simulink model "DriveSystemControl"  (R2025b)
settings: Solver=FixedStepAuto  StartTime=0.0  StopTime=Inf  FixedStep=0.001  RelTol=1e-3
PostLoadFcn:
  | if any(exist('dsrtsu_mdlpostloadfcn', 'file') ~= 0), dsrtsu_mdlpostloadfcn('Execute', bdroot); end
InitFcn:
  | , if any(exist('rtifpga_mdlclblib', 'file') ~= 0), rtifpga_mdlclblib('Init', bdroot); end,
  | , if any(exist('dsmpb_private', 'file') ~= 0), dsmpb_private('dsmpb_mdlclblib', 'Init', bdroot); end,
libraries: dsmpblib x2
(part 1 of 11)
PreSaveFcn:
  | , if any(exist('dsmpb_private', 'file') ~= 0), dsmpb_private('dsmpb_mdlclblib', 'PreSave', bdroot); end,
CloseFcn:
  | , if any(exist('dsmpb_private', 'file') ~= 0), dsmpb_private('dsmpb_mdlclblib', 'Close', bdroot); end,
settings Model: DSRTSU_INTERNAL_RTIFPGA=210  DSRTSU_INTERNAL_RTISTBM_VER=23.2  DSMPB_ID_DATA={'1682',struct('BlockId','6bd650a4-7775-4d86-b31a-c7f0cedf2a0a','SignalIds',{{'4d2bf920-403c-42ab-9030-2d9a518b8196','082edb1f-c2f8-4665-87a4-209449b9f104','8d6dcef5-afb5-4d9c-8807-a0699477d6a2','696e1246-c3e5-43ef-a482-7f0d2a84e469','04ea9c71-20d5-491c-a4d1-bb4739dee859','22128026-58a0-4e91-8829-95262852fedc','d869dca5-5dfc-4333-ab53-b3c3e836673b','bfda82c1-d835-4bf2-bc95-aa6ac6e5c40d','fcd5dec7-5735-4e3e-a193-55dd29f5c2ca','a956f46d-fc02-42b2-939f-52e903401f84','ba0c140a-12e2-4a57-8f34-0febb42557d9','6245ff97-b87b-4a0e-8af1-46c4fa2f7fc7','f1293028-aaf4-4ab8-a6f3-082efad6de70','4507e507-dc38-4f83-923d-a5bb48766b92','0dca0241-a3fd-4e55-88f7-513605b5dfba','834a7716-90ef-4018-9252-7e4f04a52069','07042789-bdc2-4e73-a93b-c580a6561b11','74a5c4a2-e22e-4a18-b0cf-773234170c76','a5f8784c-5e53-4949-bb13-5d4dd9b81511','b86019a8-98ec-42d9-9058-f7d65ce9bc5f','188db015-d143-4b34-8c9f-82cb82752dfb','366bfd7b-b2cf-42c2-bb64-21f649b82e17','56ce3dbc-22e3-4204-9c02-f638be6e34b3','c5b56939-1f0a-45a5-9add-669c4c1c62a9','1ad4e223-a404-471e-8730-84e482440c78','9e360379-29d2-4068-a30d-e9271ebfc388','f3f3b8c8-541b-4139-bbd6-2a1bc7723500','32ca3840-ec13-4611-92fa-9ad8c5b7071b','be90de92-4fef-46e1-a0c9-0c40f053aa9c','ba7c0e19-3886-43f1-b27c-69c8bf345196','f9a9b832-0eec-4c32-9774-a7523f529248','e45c8cdb-1cdb-422a-8410-eddd01433567','a79a95c2-bbe1-496d-af6c-65c2c1823672','9c272c79-fd84-4dfb-b005-4b36d7211f30','65dcbbdc-ed0d-47d3-86f1-005a976d3825','8cd805c0-b5b4-4a60-b130-463abf004e7b','a92407c6-04ed-4db1-860b-a24df70c9f97','35edea2a-57c7-420d-aeb3-abf130676984','687fa54f-b94d-448f-a202-370014edac18','b66ac79a-bf51-482c-acbe-a3be231ec044','b493fc17-940e-401a-9995-4d5744c4b1c2','c60e8434-81ec-43b4-bcd5-ce3e34bb3ef5','7ee8398a-2983-4478-ae8d-4ce734bdc1c2','03e69da6-cac7-4a63-87c3-86720c025f4c','48314e02-3fbc-464c-9d90-00d050306e9c','265a4ca5-0bbb-4b38-bb2a-a2c08d6fca1a','83cdc130-4833-4e41-854d-088457fc960a','1416cd66-4df3-4e4c-b187-45789655d8f8','76ad3dbe-0da3-4522-8c5e-5474070f195e','d1ee8ec1-428f-4fb8-83ab-9e5ead026dbd','deea3998-c4d4-4a25-95d6-c2dc6682a3e1','80711744-f146-4f9b-9cd6-5894606187b5','0090809d-e758-4f68-a9f8-fa40a0cf78a6','1ad27d01-33ad-4ad2-8310-e10dd81bfd4f','9ab4187f-c415-4d3b-862e-fd145dc08d78','7ae8cbda-f011-4195-a5ba-479d10d6282b','0d660bf5-2e1c-4ac7-88f9-9e6d591a8ce2','b955299d-9be1-46fa-a0f6-87c26013018a','16df8238-600d-46b5-8355-2ebbc49c0509','0abd2c88-22ad-437b-b7c1-aa302cf4af2e','3837f3e3-7da1-42f6-bed2-e741816623a0','4bcf49d3-b8dd-4420-9e43-0fe41c576929','e41ac73e-d8af-4fcf-96e7-9c28cba251f8','b42dae81-8c8e-4813-bbb5-2f39e8a2b7b0','34b876ad-f245-49b0-b8f8-6ec682069e3e','0c98834c-32a8-41e1-87b3-41f8c1525f50','f30d359b-60ed-4c16-aba3-c6dbef863c96','e9962dc7-0d51-4704-b146-a250d37b715c','f34f35d0-b2c1-4cc5-bb55-4c89c3895b20','3145f379-fcca-4d2e-9002-7bb4c684f0a2','a8df7938-a0d0-4f86-87c4-feca9f5a4372','efaa0a42-a334-4454-a458-d3ac57d5c708','dbdc91b7-596c-417e-aeda-55eb1ac9396d','78b6fff9-505d-4b83-bb79-dadedff90153','7f2d90e7-a6af-4e4b-b796-bf3eabad6eaf','4a0f3a51-4b5d-4063-8cad-a0c21593ff21','e7d20947-3574-4b2a-b795-fb92de4815ed','cdd8f3d4-c4cd-486a-8349-9e1c4ac1a441','555fc523-09f4-4d74-a313-07337e384831','4373e4b1-a00b-4605-aae0-5a5911c23d05','d23501fc-251d-4c29-9393-eaf2c32577b5','aa373a91-4704-4261-9894-f6d5aaf800e2','3c39687b-339c-4d6a-af4c-ad8ecf66fba3','79c9f007-2a19-4611-9c3e-2f6973c0894e','d0c345e3-cd96-4d07-931e-77de4ee97483','49d05b07-b31e-462c-b069-bef8e78563a2','74c9e241-3b39-460a-a122-3519498ceecf','06c0452b-9086-4544-b0ce-aa65222b762b','642581db-1098-4d76-8c8a-ebe9623c49d0','500df3b0-36ad-4b2f-8668-c76bfdb5893f','ff5c5439-2267-4b03-8489-22e5a4527a7a','7f70c939-3038-426d-8a53-a5fc3ecad7a4','f8fd3f50-678d-45a1-90c1-14f8a7ef1f18','f9deea20-af62-4f3c-82be-ea4cdd79cf17','16b84725-3346-447f-9fca-e927ff9b97aa','97121917-7375-4966-a993-77978f9545a8','1ebc6d63-f4c0-4836-b6a8-cf94f8c40ab6','7469b1b6-380b-469a-8ddb-87dc7f11f4f3','fecfe079-c049-493b-8842-df4524f19acf','30157484-4fb3-4404-bc3e-626bd9022609','90c29c88-b6bb-4df2-ae3d-dab8302c7e72','891d6475-5f7e-40a7-80d0-0faf1364944e','ce6e7f2b-cb3e-424a-8b0f-3ef4d0f778c2','80a6d053-d3c4-458c-bdb4-e8d2f1d58b6f','f5d19550-38c6-4cdf-9d3f-c7ff2c4edf42','8679dab3-89b2-4b8c-972e-adb9b0956be1','6d1a9255-21ca-4408-acd5-50988fe8969c','51dc251d-1242-4cb7-b761-fee981f77b9c','62132aa5-934d-47a4-aef4-8ce71be6cb39','54be5f98-a02d-4a55-91b7-e0eb3db5b29d','42ef34f8-decd-4543-af15-90924bc8905d','c9efaf1f-4082-4ddc-8e56-c65a017542cc','48f0e1b9-c04a-4854-91c0-35f6c82faf8a','1f3eded7-d459-4795-8dad-7f0dd28c087c','8099e6fc-762a-4979-bd34-a91a25cd7676','3527f9bc-ed9d-4dd1-84d3-55a707f8be99','1bcf277f-c8d2-40a1-8315-1aa473223f2e','fa6c0776-aac4-48f3-9396-764daca02d47','8387cd85-a5c1-4904-876d-f704e78f2c62','387533fb-e797-4ede-99ca-d4db8180f387','1c4c3dd9-5635-471c-935b-5eec6f46986b','e459a777-4251-4b7d-893b-90ad6317f334','17defb02-61c3-4cac-8487-2282098c4bad','962847d2-edea-4051-af97-97b08626d83a','42a313ce-3314-452b-ad2f-f3a113c22cb3','75d3fcec-c027-4b3d-bb70-d22582f25c13','fd2a2273-8951-47ed-835b-df74cc3ba1c6','bddf05ea-74a8-4d40-87a5-fa5bd6bdf322','2fed9884-dfc8-4a84-ae8f-f244653a61d3','9c3f887d-4bcb-4f6c-8796-249e51e8bb68','959b4826-76d3-4fc3-a833-b714fc953f9d','e7570022-f6c4-4e8b-a861-bb6066ff821c','b83962a3-0493-45cc-9bff-babc028f8765','1c359195-adf3-4f7a-973a-0a2c48996ddd','b2deb9fa-fd3d-4fdf-ad07-8606d6acaf75','88712765-a778-4989-9373-32db34a7e96d','3e70b9cd-2371-4f82-b9f6-12ee1415d8b9','7d58b90d-1048-43eb-af67-3288cd86feb8','01444fd3-9787-4cba-b0a2-4888be12992c','9db5b754-e9ba-4b7f-8ca9-81a8af447387','bb3c8869-bfbf-4ea7-bad8-83df8fbc8f98','5ed3fec2-9b08-4d98-a442-0ce35e27cc88','f0712c27-75e9-4f86-b8a8-ba457760ea16','5358583b-35c4-47cb-89a8-767083e8d807','023bdaf1-a030-43b0-9700-cb477693c83b','8dd5c8ed-0ddc-4ed2-bc0d-28f253869c67','9c9da58c-c166-4097-b5fa-7ea9d6f6695e','dfb39263-9b69-4474-b81a-c4d30d70140e','ccc703b7-f3e5-4cb4-b5b1-83ba1caa6f6a','52fe69e6-650a-4d77-a362-9076dc4ac840','565d162d-d064-4790-89b4-314f96e2621f','0ccdfb67-d94d-4e1e-b614-260b93448974','f50cce07-cf3e-4a8b-9eeb-7142a34334e0','11b69825-057c-43f4-9a52-cb286eff8a67','d1d74e82-881a-4d6a-99e4-eba536a09dfb','2e87cb75-a918-43cf-9a95-f0e5eace9422','1fdda0ec-b29c-4da8-a1ff-2f579d2fb1fd','4e5165ab-f934-4af7-aaca-f8701864098d','3f448d55-1dba-4c7a-9308-f0598cb6fa01','afead3bb-0504-4425-9c8e-ad2a378fa778','2fc7a59c-fc8f-4fcc-b5d5-65e69e44638e','435b3590-798d-4988-8dc0-ae2dfe9fa36c','4ca3d702-9700-4467-8bc0-5ddda41c78d0','744d85cd-5be3-4dea-a3a6-0064f59251b8','d914b334-6d5d-479c-97bf-c042d637b381','c67e1c2a-0e05-4b9b-9862-c5b24a3e52b1','a8bbb01d-de2b-48ab-82c1-4010a7c7741a','69f9f471-42d7-4015-b2e7-5a903b3d223c','6865599d-3bab-436e-b378-8a6065ccd8af','228dfb07-2cdc-48a2-beda-1fa90fce3f7b','a8fc89ea-6636-4534-9ba5-5ff0ee9f268a','f6fda9d6-d985-4630-b1e0-efbab3a7f748','0aa2a0fb-9f0d-4277-83e4-df9dffda4f6b','045875c7-e102-4128-bbe5-63fa3b05832c','cb5cb840-8ae6-4f96-ada0-a55d4e4d95ce','9c81d51c-ab73-4745-9266-3acf8ac06247','e4bfa2cb-97c3-4fbb-8dd7-6355edc7a0f8','713cd20a-a3f2-4ba6-88e8-80a6ce871d68','66ee43ba-5bdc-41d6-857a-0f6935ab8e39','13292625-30bc-4997-9e6b-497de6cb1190','acd60d88-547f-4390-beef-35e3f10afbf2','06cf514c-8df1-40fb-a85f-61544231c781','3335d807-6857-4b5d-8713-cbb5aeb56245','8263c7fb-fc40-4678-904b-dfada2e27b25','b93b61c6-d2bf-43d9-8ed3-0ecb89309517','ea82cabc-8a5a-46b8-bb1c-22b49babb383','5fa73027-c1dd-4fb2-892f-8bca7fb9b94a','82f31a19-c2c5-4607-989f-7586beda9dad','d76ef0e8-d179-47a1-8ca8-dbdf90b2a140','d501bdd8-1a03-4416-88e3-6351e0c46002','993ca02b-e763-4089-9f78-884932ce66de','b96a593d-cca9-438f-bdb3-641fabf17218','7558054b-8ba6-4fa7-8754-04b15e84ee6a','d7bd8e5d-2ff7-4dd2-bebf-c2bdb021b32a','94aa826e-0097-41c9-a4e0-cc5dd6c74607','c03f5656-a05e-4c14-bdf0-c421ae208cbf','49f7be12-6ad8-46f0-8a68-95fadeb165e7','2ae149b9-9578-4644-b4ce-ddf2e155d9f1','d6938736-adca-47f8-89a4-0915447342c1','cbd99736-1323-4b52-9170-d05d706ca95d','917397c2-3823-4180-b1c4-179169db1045','bbd7391c-67cd-411e-b5f9-3ac9dbfdb24c','7dfd2c75-dced-4705-a5e9-2a2a2d4c1ed2','85c981e9-72f2-44e5-8699-e41a8b3df25c','dd72fa7b-e733-4fbc-af40-78ba69e4bb53','bc0cf145-a984-4d25-894e-5a8c07d2e8b6','8918bd77-24ca-406d-81b0-9f0f71eaa5b3','aaf49a73-eadb-4988-9e1c-1f4687a0c5a7','88db5271-3e64-488e-8998-db478282d9d1','5d6ab81c-a00a-4771-beea-f142fc88acd1','46b0c3f9-c34c-4232-a295-52e3606efea1','e47f8773-eb71-4d5b-973a-54a731f551ff','085e50a1-1138-45fc-a57d-5399a02ce4d5','a344b347-226e-45f1-b0bf-9cc140041033','90f24455-1319-42d1-b784-e412caf3a4ac','e2e9fe19-b98b-4af6-85dd-ec4afb81798f','2eaa310f-fafb-4421-953b-c578c89e6b62','893ed9ba-a67f-4d2d-8513-ab44da56141a','7611d5a1-03f3-4973-90a7-64cf3237b486','3ae57e55-9b3d-409b-a7f6-de24e0e54807','c32b3135-c5b2-4e6d-a033-f1d56d13b3aa','0df06ca8-5346-484a-a408-79d691d949a7','5c9a9b92-4eb5-40d4-bb24-32f8ca60fbf2','ba01591a-99ca-4f3a-a480-0b29c9493ed5','2be9e2fb-4140-4463-b738-10266a35bf3a','615d2e04-5e5c-4153-a094-c8ec447c30d3','55a69a7e-6023-43c3-b133-bb865a033567','f9bc7cf0-32cf-437f-b915-b91298c7960c','43dc8092-f3fe-4614-a6e8-4088139e8bd1','b235cb9b-c3a2-41a2-85b6-9bddb082eec2','a64dedfb-6ee9-4a4f-ace2-09eb0ee433c8','f640fa21-cb84-4772-a512-7da12fd1a438','40fb2d7b-d7ac-40c8-98c5-b3c8732c033c','687755fa-7e4b-4908-a181-5af136a86154','4529d789-9ef9-4983-8bf6-7cf797bb40d9','dc2e8884-fa4b-4ff6-8f58-4e5e018f2bfb','3f263054-263a-4fa0-8fd9-a8cfe8c07787','0cbdf9b6-3173-46d3-aa7f-08b1c97744df','62cce852-fba3-40b3-93d8-491895877bec','cb4b3a9d-4f04-46df-b3d8-4697ff999350','ce6668e8-c0e7-495f-b37a-2f268e9d531d','85245983-2e26-48c5-a724-bde71d713a38','4df0109a-d5c5-43cb-8227-843af0b156a3','7ebc83d5-ad1c-48ce-a6e1-c6b0ab638476','5f64f960-7181-4cb4-9b5e-fc8b5295f45d','41fd1b04-a66a-4364-b9db-6aa7bfff160b','ea3e3dd4-c3d1-458d-adee-604f83a1ee04','af992076-6822-4ada-80e3-ab6dbc5d9d4a','c98eccdb-4c6c-4db6-acb3-c038b733bfac','ffdc664f-aa83-4dff-8e24-22198390c623','8887eef6-f5be-493f-8399-9f81aef6b3fe','a3528d63-51b7-4ac5-9b90-dce70b5af3b6','ad3f5d80-5856-4ce3-b36d-eed9eaa3efea','00c26369-2aa0-4cad-a24a-1697bf176f97','31b89546-fd4c-44d9-b714-de647cfcd9b3','7c80e928-01e1-49a5-96ea-91f6f9f61a2b','ccdaa406-b4d2-4ff3-a2f5-cf4e1644c887','2ae4ebd2-73d2-454a-a6ee-b929d7cd9a6f','4c7480a6-67ab-4b7d-b1cb-8e892c1369c4','b0d7b28d-4bed-415f-aa8b-6ae9d75690f6','e8908c6c-abca-4b58-a419-5e9c3e02e2e4','add271c7-7c49-4768-ba7f-7043464bb221','2470019e-d8f7-421d-8a57-7a385a3d6780','6f5bb2a7-60f4-42ab-9dd5-034207f55142','f911aee7-c5e8-4e2c-83c8-defc6b1f5653','38f16109-5af3-484d-a1aa-bbf2744b3099','c49c3c33-831b-40e5-8613-00f9b6836ba5','9f2e7427-64dd-478e-907e-1bb111fb7334','7eb8d7bd-f8e4-4dcb-b36f-c37d8c5e15d7','1b3ca147-0424-4ed3-ac05-fd4715a7f247','3b9bf52a-173b-484d-896b-4eecbff99b70','5f5a62bf-9d15-40da-812a-293289ce1b56','6d87a8f2-96ff-4bc1-bb1a-706893b7af83','eb9f571a-4bfc-45bc-aafa-e339e141cb62','b024688b-8b72-4461-b70a-62d23389103e','d6ced81e-c41f-47a0-9c81-f2b18ea1e2b6','7563f16e-4634-4ab8-aeba-4bc6beebcdfe','4ab347d0-3229-43f8-95c0-de0104dcaba7','2f90c9b2-549f-4e38-b380-4a5c8bc2e0b6','504b50c9-25bd-4815-ab13-0da8bdb25c30','3c742c5c-b08c-417d-8795-0984c0333b9b','b5e99845-aa43-4fde-a8a3-234b17d30c19','59c0f048-8280-4d2b-bf7b-44fdeb4866d2','824bc859-b681-41fc-81b4-03ccbbbc3a8a','77731384-ba52-458b-8862-31b6aa2e9195','38fee5a6-2ec2-4c23-9671-ad9db19ef98c','81f68cdd-f880-4766-9962-450b510dca2c','e36217fa-72f4-424f-a1ba-26c56e3b9a0d','f68425fd-7a5e-4827-9af1-d350a4f38e36','6ea8ee41-3bc0-4644-ac9b-1f597c99a9c7','ab82a394-39ff-41de-a9f7-cb5ef0534498','4f10cdaa-3e15-43d3-8f79-6b8dbc1a7a38','522704e6-d62e-42bf-ba3e-a117b8a59b5b','e0a877d8-8871-462e-8559-bba47ce65c7a','1046ff0a-d910-4642-a4a6-c04fe5f52276','6aa983d4-51f3-487a-ab56-90ed78ca5151','24efa16d-19e5-44da-88be-4fe7ecef26c0','81f68b0c-bdf1-4e45-bfd7-e55567c3dc04','4116bf02-b21b-4eb1-adf6-3e3c0dd2eaf9','6066ab77-e5c9-4ec5-b285-858f37379a7b'}}),'2',struct('BlockId','fdeae165-f251-4e82-b59a-3c43838b8ed1','SignalIds',{{'de8b44b4-5422-44ef-8723-6bdca849999c','7b06e3d2-1eb0-49de-940b-866532a21950','74468e4d-ce7b-4114-abcc-ff4ed516802e','09b3dc75-925f-4156-8fba-f27b88531e74','0d939a05-4c0b-4c2f-ac9f-c224cb75ad55','61fa365a-d2fa-494d-9414-3405a4ce6d0a','ce00d0ab-86c1-45f0-9867-9a3821da710b','f31fc571-c561-49d2-9f91-922cc8d9329e','0a751642-ad47-47ce-8c4c-87b9c8bace46','b29db070-bfb7-44ce-bbb4-dac7cc04df61','a0b6132c-c02b-4ec6-93db-95c6745521da','d513a490-61fc-40bb-9b15-a9912397190f','5d11f126-fe30-4254-9ca3-30fe71e76f3c','48fd1300-cd08-4009-87f3-302b4ebf7052','66062813-008c-473c-8e52-deb424770f9c','e0ce1efa-3209-46ec-8e83-f1336c285641','2f9e3794-b3da-4bfa-984d-30fae498b990','83f662e2-91a8-4716-96cc-1d31ae3903e5','ed013d79-9480-43d1-adbb-ef641568d862','245c77d0-9eeb-4469-8ad7-ddd6cca0bdc7','109a2097-3c50-43cf-b22c-e32e4f0d4b16','5c8654f8-c4bf-4464-ac59-550e46dfbe36','053ac246-b2f3-4500-b8dd-d680c86b03fd','7a8feb55-fc6b-4238-91ea-6e4b4e7558e7','d016b082-1aa2-4773-a812-75518ae20876','8789bb0c-d99b-4489-8c7e-d41abab79294','1b300131-2ece-46a4-ae79-1cd046174832','27185aed-9b16-464a-8e1f-1ad039b150d2','dc5d8b8b-96a3-416c-8c53-f6439024a3f2','53d4b546-2e80-41d7-99aa-9cd9e4df08a4','9d062d5d-415c-4501-a210-a13c9dc09661','f2802ce9-2474-405f-b2fa-9033a0c19371','c35b0d99-e3ee-4fe3-adc4-cd41e3c76d9c','2cf185fc-7a78-491b-bce7-d7593e39c21d','9f8b6ee8-2ea5-4f6f-8f38-bdc62e5a5876','a5d2abe3-156f-45fc-8d82-5f1c828eee06','60f59446-fa5c-4a1a-9f1b-2da327279d46','8f11fc00-2091-4a34-8c6b-ba6a227f3728','b48f3cb0-dfeb-42bf-83a7-6d2e2c9f28cd','df21d149-9261-4d80-ab0f-bced706a3188','b57734b1-8e0a-44d2-9318-0d83da79d543','6faafaed-af4e-43d7-9806-29c97c255c6c','233beed0-43f0-452c-aa34-82cfbd4d48ac','465d0d2b-5ee6-4937-9a44-db7d6bb66479','bc7ff652-41f2-4daf-879a-5b2921b89016','7c3d8010-5c5c-40e3-b1ae-5692f53c86e8','9666030d-3a17-4d78-a81f-8b72e34b0b66','0c513926-8004-44fa-98f3-f956c2aab0fa','9166d83e-c4c2-48fd-b219-1b7c9d6557b4','cc755fdb-0eae-43d7-8eb6-4ca175b2ce2f','bc3a07b2-a619-4c81-b3f8-feb17cfbcce2','4e564945-a3a3-43c1-841e-93b5d941de79','09af9a1a-9f3a-490d-a22b-1e244a520192','0fee6cdc-ddd9-4de0-9902-dc7f9d2495d1','cba0aac5-3610-40ba-95e7-3214ee2eb255','d957393b-e4d4-466c-8db6-61d28ec803fb','d8a45f3c-0399-4f7b-965f-ebd23a625cc9','74696636-2799-47bd-b6c3-7bbc02a97467','32df2c93-5398-4279-82d2-8ad464d076a6','45e3dc24-a076-40c8-938b-1c108a74d5d1','735a660d-7436-48bb-be5b-89cc0edc3658','10980fb2-941a-41b9-8141-8bdc6fe828f5','4d8ae5ff-336c-4f2e-bd45-d0e31a4eaae7','955c6127-9ce1-461a-b6d7-5551c6febfc7','522dff20-4a47-4e98-8115-6a9305e6acfc','c2400870-07cd-4018-a99e-23e7da5108e1','75701347-3308-45ba-bfb0-7d593a167a16','5b1f0e37-5598-4687-9cc3-c7f1d3495d80','b355af3f-48f3-42fd-9da3-9c53df86dd66','84090b07-4cf6-4aa5-a80d-19288670be82','2e4363a3-2349-4f09-84e5-00ca8294403d','468f28a3-7f8d-4e9a-98ba-22c9251e9022','b9fa48eb-8926-4a45-9a4c-2df5a61da293','2e70f4ff-309e-40ea-bc25-5b9c3b09de05','19980cf7-9fa9-4830-9d3b-932aceb94898','7a57d7ac-979c-41f6-a94b-75fe1c9dc488','4817d061-27af-40f7-bb85-993186cfface','7bff44ec-3940-4df6-906b-5ebb1cd609eb','4da95aff-fd17-4a13-ad0f-df6500b75cb9','67be5fde-06d3-4a91-b8a8-8f5a874bffb8','aed8f512-8d75-49d8-97ba-7cdcaa4ec92b','2081fd6c-66db-4b19-9031-a92910431a1b','9b269a33-7c5f-4e87-8838-4dbd5e03684f','ead4c6b7-092f-4771-98e3-f228bc0df61e','09d15870-e3f7-4818-9260-8cbd79fc4934','e1c4632d-8d1d-435e-9cc2-1a1d7cee0134','be392e74-2c9a-4303-8deb-b6ebecb41bb2','3d160701-0a0b-4a9e-911d-7e5f1dca8da1','a10638db-8be5-418f-90c3-8a20284ef010','46845510-bea5-47b6-a852-33e47d9a4bbb','1096f6c8-0051-4daa-93bd-08ee419c3d60','e40a998f-3667-404e-a490-3cb0f0305e64','de91afbc-364c-4d90-8544-7e581d5e6036','977c9308-4cf7-4ef9-9655-eecccd4e37ea','8135e324-4d45-41aa-9edd-83d48a353d7e','cff61663-a888-46ad-8242-c681d34892b0','c59df38c-1b9a-420d-b5b6-7b02e9f30d14','8c3f161a-015a-4ad0-b6cb-70b756673a80','ddea31d3-517e-4adf-adc9-8410399cc30c','2ac0e3f2-35de-45a3-97da-d45fd9866c6a','5cf57e47-2f74-4e53-be91-f6f7c6319c02','e6ebc12b-6c7e-4c2d-89bd-1e13fbfe96c1','bc7606f6-bdc9-4d7a-a134-d3cf085f353e','652e12db-6510-47c5-9cee-3289bf08fb81','32dcee06-8d73-4567-a14e-b4948d0c7c57','be60a994-383f-43e0-a6a8-e25bbfdd91de','990e0621-b375-4e80-9796-4e4ace91b209','bdd403ee-ec2d-44e3-afc1-6fe71c0e26eb','81afed3e-a265-49a6-b3ad-6cabe8f91ecb','0a983437-82e0-4732-bd97-f41efdc05314','5e76d710-901b-476f-954c-5430facedaca','3be0e1ca-d6bc-4bd5-b8d4-50e1289b089b','c504ba16-f24b-4614-ae03-4e76a49f7adf','932897a8-81cb-498b-bb33-ea7d7b0238c4','f2665638-91ea-466d-97d5-d52c7b16d6d5','043e2de2-04fe-4e3b-b0c6-5ddfa18c1d18','8f3c1a59-5ef2-4f4c-9629-a0484fad656d','2f116884-4cba-439c-85c4-3547126edc4f','dd612bf9-7c57-4164-a759-b3de7707c278','4b187830-e30c-4f4a-aa7e-32f00e661252','fbf0f747-84c1-435a-8184-a67b43aa0379','b3a9ccbd-8fd1-4c1d-8fd1-4362dcc93e97','f6f40c37-99f4-46df-b3d0-72f5d2793989','1ab4b575-6948-4afe-9774-20425c1a8951','07728060-6cc8-4bf9-8b9b-5f5596c45ab9','ac6d2f26-54c5-4a67-bbc5-680bf04eb5d8','57e3ba4b-9507-4f5e-8ed9-618e71123933','de0c428b-5ba9-4ad2-8078-206528c55396','afa35936-e8ea-4a9c-a9cd-c56e07d7689f','0bb38e01-f1da-40c0-a9e9-6de8e14cc2c0','47a2144d-6aeb-4d86-bd89-49b5844ec041','65b96597-0582-4f2a-86b1-26455202c868','ff25c3aa-f958-42b6-9e59-f5a026dff9f4','2905a61d-4f68-4d1f-978a-afc6c65f5737','3a41da83-63a1-46f9-a952-8b9af7794f2c','d5d01b3c-f436-4b5b-82c1-142de6ff27ad','447ff66a-31ed-4fbf-aa67-6305ea65f05d','278a5484-cd16-47b1-b117-efe68225702b','5c3ba11a-3515-4c0e-868c-f2cc44378a3c','b8a1b769-223e-491b-a256-ec5a6f28fef2','a1d96fe5-c3ba-4a23-901f-02173da89a20','4b9770e1-7a75-45a9-8578-d72916c107a1','c27f1bab-f8f0-4a84-a154-2f177810a256','476fd6db-b212-4592-9a4a-c22e7d6b84eb','2e4e1afb-2734-4baf-97ad-0100df7323f2','0210cdd7-b46c-4281-9a52-c0544873f54b','56144df2-637e-456a-ab58-3430fca16b2a','dbfd772d-d01c-48e7-aa6b-9e74b92c9a19','61bfcd02-3e15-4f08-9ad6-0a80ec366a4a','d76c8ffb-b399-43d4-bd45-30aa88148c11','3e57bbde-eeef-433a-9c1b-4ff6b243bcb8','ecfc6bcf-12a2-45ec-9ee5-91807b0ae174','32c4bb39-d309-4ad3-8e1d-d33ca5046e76','7846b9f8-0593-4e8e-8339-59be79bb9e44','8c280d6c-ccc3-41c2-aefc-75b0b983aba1','b8245033-a011-4e70-b677-32c48ba319bf','1806b3b9-7fa6-4329-aad0-38a4cc9c3a0d','3cc78dfb-37ad-432b-afb6-10d890ce3613','a580af44-a49f-48a6-a1e2-bc7cd1a7761f','7eed13f3-b9fe-4789-a07b-330ca8d35faa','93f81d31-f14f-4bc3-a614-8c0b4085b5d9','73f1cef2-8057-48cc-aa1d-ac1323c43fb1','5db861ba-aaf6-4c67-b7b9-bb818399091e','e7ee0ff6-14e9-40c0-8ac9-4df9f11a6683','bb839128-0c40-46e1-9127-4d997c649eba','f5e2cee2-6f4a-4069-8698-01e792f15bf5','040c843c-0881-46b9-8ccd-7fa67e5a8526','a96a21de-c0f1-480e-abf4-c62a0a739262','0b64d65c-92c7-41a8-8fc9-f7ccb397cb14','9f05ec84-b3f2-483d-a38f-5b354dd2cf57','480e317a-2597-44d3-8213-8e3d613866f8','24b4c2cd-7e82-4de1-a48b-a7c044870a20','81966acd-aa96-48c8-8018-a9545624582b','2c2af29c-d3e1-41db-ba0a-1f865aefb512','7c0b55f8-ea91-4077-bd8c-cc6bfb22dedb','85588d04-f050-4133-a21f-7692b804045d','107279e5-4394-4265-ab5c-29a6df39d858','10acbf4c-799c-4e13-a154-848ef2cf3d06','10dad0d3-d666-4179-8b68-aef958647a07','5b8c799a-4e30-49c4-8ab6-ecbb26938cc1','fbca3a12-5897-4410-bccd-82575ad7b2ff','529fcb8f-b307-4514-9620-e1b2c833d4e3','067906f9-22eb-46e7-b210-dcfd1b0b7eca','1d8d3c3c-58bf-4331-b897-e4eafaa5b8dc','03c82172-e26e-4cf4-90d5-2195b8000227','655349db-53c1-47fe-9446-0ee68c443f65','2e018f93-4293-4832-b3cc-e4db5589e226','147eea70-4f58-44d2-a21e-44109cd1bcb5','66945845-1ce9-496f-9a4f-ffe4e51837b5','499c724f-c37f-48ba-a1f4-28ac52df7ea5','b6794d06-edc0-4606-a429-57aabafc5ce1','cbc1cb93-8de4-4a68-81da-eeb179512be7','63184478-25f8-4e5c-96ab-f649643fc6dc','1d4d4c13-8d7a-43a7-82fa-8823d056fb47','a7010fba-113f-4abb-934f-a1d598db6650','d60151f6-e2bb-44d0-97f5-b9a6b446749d','c6e18689-1cfb-4099-8655-dbeea30a1865','bedecf49-055c-4280-a56f-d9cae2990382','4f1ce29b-2afe-4ca7-9a57-22a60e90ba30','94c28d1c-303a-4304-ac13-44f231e8e68d','59ce40cd-53ee-4803-9e0d-e5ea17f4cff9','9a5167ea-a9ce-4bae-83fb-71637c8cd1ab','7e45628f-bf64-4921-a76f-4f974fb9fe40','9b3f5dfe-9eb7-4a31-abd0-56a510178dc1','75cf1272-a273-4083-a26d-3fea507291ff','0fc378fb-3d88-4771-a129-17a736f54c2c','b241270b-68f3-40d1-9491-2ee7e36148c0','a769bb7d-1d78-4ec8-a3f6-bd492bf63750','576bc8fc-bebc-439e-b4c8-3086d4f4d778','e0b9c0e4-0e15-41c4-a55a-5c8af835c3a8','7ce844ea-f31e-426c-bdfc-26589907def4','a94b0dab-8855-4ff6-98fa-d5b0fa5f7cbf','5e2634c0-e882-44cb-af7e-da85caa29e0c','2f4703e9-16b6-412e-ae5a-daa5147d0e99','9df47e29-c871-435f-b6d7-9bc6a45234c3','0b7e4c49-dfb8-4e4c-be51-2aa0924f5d0e','30848cd8-b7c2-40bb-88e6-af4923ef4463','803dbca7-d9d6-46f5-9b8a-1f5dcadc40ab','8276e255-0345-4bba-984f-28286ab88662','2e1dc2d9-db99-4c3c-94a2-1d1accf58fd4','bfbfcfe5-c032-4f33-98b9-f08a142d4b3d','2c76a0a7-75da-418b-92b2-b4abbe9d7631','3ee28d08-8b83-4b2f-add7-3a450c57c357','edc7a7e5-1201-4829-a751-479dd5624d67','22440fc5-d4b1-4a38-af36-e4aebaff63cd','4e8cf599-944e-4d81-a460-d342d6d656bb','67187d27-f8ae-4e07-bd5c-8f8e68ce107f','31813405-b512-43d5-a107-22f42c7efcdf','12a3c7b2-0ef8-42ea-b257-433533060951','94d7e6c9-1a49-4644-9642-7d23adffa9a5','41af8ef3-86e3-4f2a-8ccd-b49473830aff','291e49a3-cb15-4225-bd5f-cf812338c3a6','6ef9c6c9-46a8-48d5-8bb0-804c08aa3838','f53d4411-762d-4469-9b83-26ad48e1d186','2c14f202-fa96-49c7-af6e-229620f8a5f6','e161c16d-c154-41bc-8151-bcd304adeae2','e491f51a-aabc-4e34-b99f-32892cce09eb','6f3ced98-1f32-4227-af27-721b08ccae0d','ab338563-17fe-423e-8c7f-6671bd4ae339','876cb448-710e-44b3-9042-04655f65fd81','cb280c1a-7567-4d63-bd86-5fd0ef4de71a','63911ff8-0890-4322-b749-398c434f08e7','14f15975-9622-4b8b-aecc-e014706ce072','cd17c7e4-da5e-4b1c-a54e-d5ac94ae44a0','ef0a9bb9-bb14-42f0-b05f-1781a6e36247','3c31f4d8-11fa-4b27-8a14-0f9f31a0fa3f','e3c1f15c-637d-4a17-87d7-3c6a9b240052','5c6aaa89-13e1-478b-97af-dfaf5001a808','6fdc1402-2e8d-4478-8717-65c6f9116fd5','780aac3f-8a49-4430-8e9e-9e74d81ed1b2','fc85fb86-64ec-459d-b0cf-9cd95bcb9d60','6db658d6-cb72-47b6-aebc-ea68633b9036','b95c7cc0-dbcd-4537-ba1b-7781767d1e14','237d60a0-3e9b-4996-8830-289ba11d6b9b','455bc271-368f-450c-a7f1-f31883bec460','47cbee84-623f-4332-834c-fd99b86fb540','79fb1432-8cf2-4971-985d-57ef54e4908c','c2795267-1999-41fd-9b63-66902f5c0d82','5f34848a-10a8-4ce4-acd7-952ff817484b','e0ae91eb-2846-4fb5-9dbd-2d8856d56dfe','fdf3638c-77a6-4082-a4be-ef4b62e07f08','7c29b997-b3b3-443f-8fae-3f9f9e1753ee','7d413e90-90be-471e-af49-f54a2a95f939','8e236231-9214-48f9-a541-987c1d5b7579','bab97780-9874-4de6-8d70-c4bd6bd05cf0','9d793aea-5988-47de-890a-db90f1c3707c','9c125b00-d52e-4fa6-8ccc-1e4806ac683f','81e509fa-0d6f-448b-8368-fb1571c0bb70','80910651-8b2b-4abc-b522-3774286ff664','17d82bd2-7fa6-49ae-acdd-a3900593374c','875b3e42-7eb5-4f2e-9c6e-b67881d72b2b','5430afc4-d9b2-472a-b6a6-0ca88bce53ff','b71a725d-0a81-4362-8dbc-22226aae632c','ce907282-1c16-482b-80bf-a6d1fed3b919','f8b9c411-1d29-4f10-a55d-9850703d42f6','15382d29-5d33-4cdb-bb58-eba90d4ab5fc','87566085-81c6-4f92-9d59-7bc4afcdb0fe','a1b5ca3d-8df0-4d46-8c07-4d1ae1986830','a4000a69-fb31-4fc4-ac92-d20106dfcf1e','bc9a8452-3b12-43e7-b29e-2048af94c161','b64bf5c9-86bc-4428-881d-5e6eb60cd202','c6ff0695-a359-4ced-9d27-40b774cacb7e','ed431a80-fd0c-404c-9126-2b84d01145b2','86d73309-2c10-4464-a04e-4b7ff154f585','923864f6-60cd-409d-96e8-3cd88239526f','394a4075-5ab2-4698-93a8-830edee76a4d'}})}  Creator=MURTI
settings OptimizationCC: BlockReduction=off  ConditionallyExecuteInputs=off  OptimizeBlockIOStorage=off  BufferReuse=off
settings DebuggingCC: TasksWithSamePriorityMsg=none
settings HardwareCC: ProdBitPerLong=64.0  ProdLargestAtomicInteger=Integer  ProdWordSize=32.0  ProdLongLongMode=on  ProdHWDeviceType=Custom Processor->Custom
settings ModelReferenceCC: EnableParallelModelReferenceBuilds=on
settings RTWCC: SystemTargetFile=dsrt.tlc  GenCodeOnly=on  MakeCommand=make_dsrt  TemplateMakefile=dsrt_default_tmf  RTWVerbose=off  GPUComputeCapability=3.5  Description=dSPACE Target DSRT - Generates SIC files for import by ConfigurationDesk and VEOS. Provides code generation for Simulink models imported in ConfigurationDesk.
settings STFCustomTargetCC: SystemTargetFile=dsrt.tlc  TargetLangStandard=C99 (ISO)  ParMdlRefBuildCompliant=on  ConcurrentExecutionCompliant=off  GRTInterface=off  DSTargetArchitecture=Default  VDFType=TRC  TRCOnlyGlobals=off  TRCGenerateLabels=off  TRCGenerateVirtualBlocks=off  TRCGenerateStates=off  TRCGenerateDerivatives=off  TRCGenerateParamValues=off  TRCIsOmitVdOn=on
settings GRTTargetCC: CompOptLevelCompliant=off  ConcurrentExecutionCompliant=off  CombineOutputUpdateFcns=off  MatFileLogging=off  CPPClassGenCompliant=off  UseToolchainInfoCompliant=off

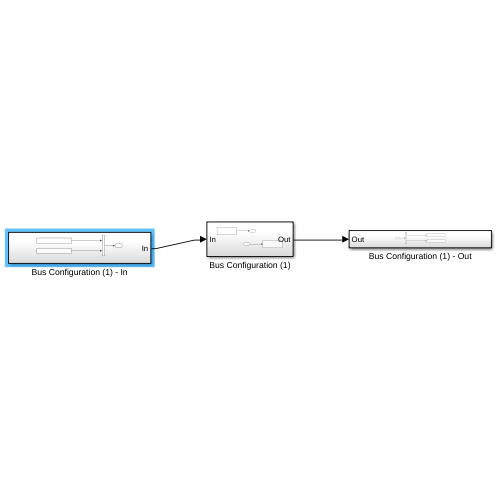
[thumbnail: Simulink's stored preview of the top-level diagram]
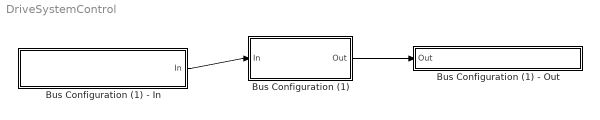
== system DriveSystemControl ==
  Bus Configuration (1) : Subsystem
  Bus Configuration (1) - In : Subsystem
  Bus Configuration (1) - Out : Subsystem
  wires:
  Bus Configuration (1)/1(Out) -> Bus Configuration (1) - Out/1(Out)
  Bus Configuration (1) - In/1(In) -> Bus Configuration (1)/1(In)

== system DriveSystemControl/Bus Configuration (1) ==
  In : Inport
  Bus Configuration (1)_In : dsmpblib/Data Inport  Priority=10000
      settings: SourceProductName=dSPACE Model Interface Package for Simulink (MIPS)
  Bus Configuration (1)_Out : dsmpblib/Data Outport  Priority=-10000
      settings: SourceProductName=dSPACE Model Interface Package for Simulink (MIPS)
  Out : Outport
  wires:
  Bus Configuration (1)_In/1 -> Out/1
  In/1 -> Bus Configuration (1)_Out/1

== system DriveSystemControl/Bus Configuration (1) - In ==
  Manipulation : Subsystem
  Simulated ECUs : Subsystem
  _In_ : BusCreator  Inputs=2
  In : Outport
  wires:
  _In_/1 -> In/1  "In"
  Simulated ECUs/1(Simulated ECUs) -> _In_/1  "Simulated ECUs"
  Manipulation/1(Manipulation) -> _In_/2  "Manipulation"

== system DriveSystemControl/Bus Configuration (1) - Out ==
  Out : Inport
  Manipulation : Subsystem
  Simulated ECUs : Subsystem
  _Out_ : BusSelector  OutputSignals=Simulated ECUs,Manipulation
  wires:
  Out/1 -> _Out_/1  "Out"
  _Out_/1 -> Simulated ECUs/1(Simulated ECUs)  "<Simulated ECUs>"
  _Out_/2 -> Manipulation/1(Manipulation)  "<Manipulation>"

== system DriveSystemControl/Bus Configuration (1) - In/Manipulation ==
  _Manipulation_ : BusCreator  Inputs=1
  gitam Controller CAN File 08082024 : Subsystem
  Manipulation : Outport
  wires:
  _Manipulation_/1 -> Manipulation/1  "Manipulation"
  gitam Controller CAN File 08082024/1(gitam Controller CAN File 08082024) -> _Manipulation_/1  "gitam Controller CAN File 08082024"

== system DriveSystemControl/Bus Configuration (1) - In/Simulated ECUs ==
  _Simulated ECUs_ : BusCreator  Inputs=1
  gitam Controller CAN File 08082024 : Subsystem
  Simulated ECUs : Outport
  wires:
  _Simulated ECUs_/1 -> Simulated ECUs/1  "Simulated ECUs"
  gitam Controller CAN File 08082024/1(gitam Controller CAN File 08082024) -> _Simulated ECUs_/1  "gitam Controller CAN File 08082024"

== system DriveSystemControl/Bus Configuration (1) - Out/Manipulation ==
  Manipulation : Inport
  _Manipulation_ : BusSelector  OutputSignals=Virya Controller CAN File 08082024
  gitam Controller CAN File 08082024 : Subsystem
  wires:
  Manipulation/1 -> _Manipulation_/1  "Manipulation"
  _Manipulation_/1 -> gitam Controller CAN File 08082024/1(gitam Controller CAN File 08082024)  "<Virya Controller CAN File 08082024>"

== system DriveSystemControl/Bus Configuration (1) - Out/Simulated ECUs ==
  Simulated ECUs : Inport
  _Simulated ECUs_ : BusSelector  OutputSignals=Virya Controller CAN File 08082024
  gitam Controller CAN File 08082024 : Subsystem
  wires:
  Simulated ECUs/1 -> _Simulated ECUs_/1  "Simulated ECUs"
  _Simulated ECUs_/1 -> gitam Controller CAN File 08082024/1(gitam Controller CAN File 08082024)  "<Virya Controller CAN File 08082024>"

== system DriveSystemControl/Bus Configuration (1) - In/Manipulation/gitam Controller CAN File 08082024 ==
  WIP : Subsystem
  _gitam Controller CAN File 08082024_ : BusCreator  Inputs=1
  gitam Controller CAN File 08082024 : Outport
  wires:
  _gitam Controller CAN File 08082024_/1 -> gitam Controller CAN File 08082024/1  "gitam Controller CAN File 08082024"
  WIP/1(WIP) -> _gitam Controller CAN File 08082024_/1  "WIP"

== system DriveSystemControl/Bus Configuration (1) - In/Simulated ECUs/gitam Controller CAN File 08082024 ==
  BMS : Subsystem
  TCU : Subsystem
  _gitam Controller CAN File 08082024_ : BusCreator  Inputs=2
  gitam Controller CAN File 08082024 : Outport
  wires:
  _gitam Controller CAN File 08082024_/1 -> gitam Controller CAN File 08082024/1  "gitam Controller CAN File 08082024"
  TCU/1(TCU) -> _gitam Controller CAN File 08082024_/1  "TCU"
  BMS/1(BMS) -> _gitam Controller CAN File 08082024_/2  "BMS"

== system DriveSystemControl/Bus Configuration (1) - Out/Manipulation/gitam Controller CAN File 08082024 ==
  gitam Controller CAN File 08082024 : Inport
  WIP : Subsystem
  _gitam Controller CAN File 08082024_ : BusSelector  OutputSignals=WIP
  wires:
  gitam Controller CAN File 08082024/1 -> _gitam Controller CAN File 08082024_/1  "gitam Controller CAN File 08082024"
  _gitam Controller CAN File 08082024_/1 -> WIP/1(WIP)  "<WIP>"

== system DriveSystemControl/Bus Configuration (1) - Out/Simulated ECUs/gitam Controller CAN File 08082024 ==
  gitam Controller CAN File 08082024 : Inport
  BMS : Subsystem
  IPC : Subsystem
  TCU : Subsystem
  Telematics : Subsystem
  _gitam Controller CAN File 08082024_ : BusSelector  OutputSignals=IPC,TCU,Telematics,BMS
  wires:
  gitam Controller CAN File 08082024/1 -> _gitam Controller CAN File 08082024_/1  "gitam Controller CAN File 08082024"
  _gitam Controller CAN File 08082024_/1 -> IPC/1(IPC)  "<IPC>"
  _gitam Controller CAN File 08082024_/2 -> TCU/1(TCU)  "<TCU>"
  _gitam Controller CAN File 08082024_/3 -> Telematics/1(Telematics)  "<Telematics>"
  _gitam Controller CAN File 08082024_/4 -> BMS/1(BMS)  "<BMS>"

== system DriveSystemControl/Bus Configuration (1) - In/Manipulation/gitam Controller CAN File 08082024/WIP ==
  CANChannel : Subsystem
  _WIP_ : BusCreator  Inputs=1
  WIP : Outport
  wires:
  _WIP_/1 -> WIP/1  "WIP"
  CANChannel/1(CANChannel) -> _WIP_/1  "CANChannel"

== system DriveSystemControl/Bus Configuration (1) - In/Simulated ECUs/gitam Controller CAN File 08082024/BMS ==
  TX : Subsystem
  _BMS_ : BusCreator  Inputs=1
  BMS : Outport
  wires:
  _BMS_/1 -> BMS/1  "BMS"
  TX/1(TX) -> _BMS_/1  "TX"

== system DriveSystemControl/Bus Configuration (1) - In/Simulated ECUs/gitam Controller CAN File 08082024/TCU ==
  TX : Subsystem
  _TCU_ : BusCreator  Inputs=1
  TCU : Outport
  wires:
  _TCU_/1 -> TCU/1  "TCU"
  TX/1(TX) -> _TCU_/1  "TX"

== system DriveSystemControl/Bus Configuration (1) - Out/Manipulation/gitam Controller CAN File 08082024/WIP ==
  WIP : Inport
  CANChannel : Subsystem
  _WIP_ : BusSelector  OutputSignals=CANChannel
  wires:
  WIP/1 -> _WIP_/1  "WIP"
  _WIP_/1 -> CANChannel/1(CANChannel)  "<CANChannel>"

== system DriveSystemControl/Bus Configuration (1) - Out/Simulated ECUs/gitam Controller CAN File 08082024/BMS ==
  BMS : Inport
  RX : Subsystem
  _BMS_ : BusSelector  OutputSignals=RX
  wires:
  BMS/1 -> _BMS_/1  "BMS"
  _BMS_/1 -> RX/1(RX)  "<RX>"

== system DriveSystemControl/Bus Configuration (1) - Out/Simulated ECUs/gitam Controller CAN File 08082024/IPC ==
  IPC : Inport
  RX : Subsystem
  _IPC_ : BusSelector  OutputSignals=RX
  wires:
  IPC/1 -> _IPC_/1  "IPC"
  _IPC_/1 -> RX/1(RX)  "<RX>"

== system DriveSystemControl/Bus Configuration (1) - Out/Simulated ECUs/gitam Controller CAN File 08082024/TCU ==
  TCU : Inport
  RX : Subsystem
  _TCU_ : BusSelector  OutputSignals=RX
  wires:
  TCU/1 -> _TCU_/1  "TCU"
  _TCU_/1 -> RX/1(RX)  "<RX>"

== system DriveSystemControl/Bus Configuration (1) - Out/Simulated ECUs/gitam Controller CAN File 08082024/Telematics ==
  Telematics : Inport
  RX : Subsystem
  _Telematics_ : BusSelector  OutputSignals=RX
  wires:
  Telematics/1 -> _Telematics_/1  "Telematics"
  _Telematics_/1 -> RX/1(RX)  "<RX>"

== system DriveSystemControl/Bus Configuration (1) - In/Manipulation/gitam Controller CAN File 08082024/WIP/CANChannel ==
  PDUs : Subsystem
  _CANChannel_ : BusCreator  Inputs=1
  CANChannel : Outport
  wires:
  _CANChannel_/1 -> CANChannel/1  "CANChannel"
  PDUs/1(PDUs) -> _CANChannel_/1  "PDUs"

== system DriveSystemControl/Bus Configuration (1) - In/Simulated ECUs/gitam Controller CAN File 08082024/BMS/TX ==
  PDUs : Subsystem
  _TX_ : BusCreator  Inputs=1
  TX : Outport
  wires:
  _TX_/1 -> TX/1  "TX"
  PDUs/1(PDUs) -> _TX_/1  "PDUs"

== system DriveSystemControl/Bus Configuration (1) - In/Simulated ECUs/gitam Controller CAN File 08082024/TCU/TX ==
  PDUs : Subsystem
  _TX_ : BusCreator  Inputs=1
  TX : Outport
  wires:
  _TX_/1 -> TX/1  "TX"
  PDUs/1(PDUs) -> _TX_/1  "PDUs"

== system DriveSystemControl/Bus Configuration (1) - Out/Manipulation/gitam Controller CAN File 08082024/WIP/CANChannel ==
  CANChannel : Inport
  PDUs : Subsystem
  _CANChannel_ : BusSelector  OutputSignals=PDUs
  wires:
  CANChannel/1 -> _CANChannel_/1  "CANChannel"
  _CANChannel_/1 -> PDUs/1(PDUs)  "<PDUs>"

== system DriveSystemControl/Bus Configuration (1) - Out/Simulated ECUs/gitam Controller CAN File 08082024/BMS/RX ==
  RX : Inport
  PDUs : Subsystem
  _RX_ : BusSelector  OutputSignals=PDUs
  wires:
  RX/1 -> _RX_/1  "RX"
  _RX_/1 -> PDUs/1(PDUs)  "<PDUs>"

== system DriveSystemControl/Bus Configuration (1) - Out/Simulated ECUs/gitam Controller CAN File 08082024/IPC/RX ==
  RX : Inport
  PDUs : Subsystem
  _RX_ : BusSelector  OutputSignals=PDUs
  wires:
  RX/1 -> _RX_/1  "RX"
  _RX_/1 -> PDUs/1(PDUs)  "<PDUs>"

== system DriveSystemControl/Bus Configuration (1) - Out/Simulated ECUs/gitam Controller CAN File 08082024/TCU/RX ==
  RX : Inport
  PDUs : Subsystem
  _RX_ : BusSelector  OutputSignals=PDUs
  wires:
  RX/1 -> _RX_/1  "RX"
  _RX_/1 -> PDUs/1(PDUs)  "<PDUs>"

== system DriveSystemControl/Bus Configuration (1) - Out/Simulated ECUs/gitam Controller CAN File 08082024/Telematics/RX ==
  RX : Inport
  PDUs : Subsystem
  _RX_ : BusSelector  OutputSignals=PDUs
  wires:
  RX/1 -> _RX_/1  "RX"
  _RX_/1 -> PDUs/1(PDUs)  "<PDUs>"

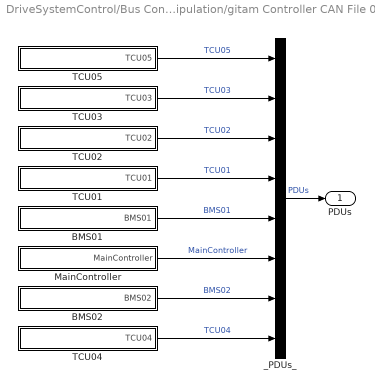
== system DriveSystemControl/Bus Configuration (1) - In/Manipulation/gitam Controller CAN File 08082024/WIP/CANChannel/PDUs ==
  BMS01 : Subsystem
  BMS02 : Subsystem
  MainController : Subsystem
  TCU01 : Subsystem
  TCU02 : Subsystem
  TCU03 : Subsystem
  TCU04 : Subsystem
  TCU05 : Subsystem
  _PDUs_ : BusCreator  Inputs=8
  PDUs : Outport
  wires:
  _PDUs_/1 -> PDUs/1  "PDUs"
  TCU05/1(TCU05) -> _PDUs_/1  "TCU05"
  TCU03/1(TCU03) -> _PDUs_/2  "TCU03"
  TCU02/1(TCU02) -> _PDUs_/3  "TCU02"
  TCU01/1(TCU01) -> _PDUs_/4  "TCU01"
  BMS01/1(BMS01) -> _PDUs_/5  "BMS01"
  MainController/1(MainController) -> _PDUs_/6  "MainController"
  BMS02/1(BMS02) -> _PDUs_/7  "BMS02"
  TCU04/1(TCU04) -> _PDUs_/8  "TCU04"

== system DriveSystemControl/Bus Configuration (1) - In/Simulated ECUs/gitam Controller CAN File 08082024/BMS/TX/PDUs ==
  BMS01 : Subsystem
  BMS02 : Subsystem
  _PDUs_ : BusCreator  Inputs=2
  PDUs : Outport
  wires:
  _PDUs_/1 -> PDUs/1  "PDUs"
  BMS02/1(BMS02) -> _PDUs_/1  "BMS02"
  BMS01/1(BMS01) -> _PDUs_/2  "BMS01"

== system DriveSystemControl/Bus Configuration (1) - In/Simulated ECUs/gitam Controller CAN File 08082024/TCU/TX/PDUs ==
  MainController : Subsystem
  TCU01 : Subsystem
  TCU02 : Subsystem
  TCU03 : Subsystem
  TCU04 : Subsystem
  TCU05 : Subsystem
  _PDUs_ : BusCreator  Inputs=6
  PDUs : Outport
  wires:
  _PDUs_/1 -> PDUs/1  "PDUs"
  MainController/1(MainController) -> _PDUs_/1  "MainController"
  TCU05/1(TCU05) -> _PDUs_/2  "TCU05"
  TCU04/1(TCU04) -> _PDUs_/3  "TCU04"
  TCU03/1(TCU03) -> _PDUs_/4  "TCU03"
  TCU02/1(TCU02) -> _PDUs_/5  "TCU02"
  TCU01/1(TCU01) -> _PDUs_/6  "TCU01"

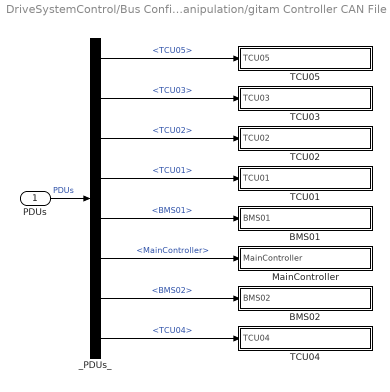
== system DriveSystemControl/Bus Configuration (1) - Out/Manipulation/gitam Controller CAN File 08082024/WIP/CANChannel/PDUs ==
  PDUs : Inport
  BMS01 : Subsystem
  BMS02 : Subsystem
  MainController : Subsystem
  TCU01 : Subsystem
  TCU02 : Subsystem
  TCU03 : Subsystem
  TCU04 : Subsystem
  TCU05 : Subsystem
  _PDUs_ : BusSelector  OutputSignals=TCU05,TCU03,TCU02,TCU01,BMS01,MainController,BMS02,TCU04
  wires:
  PDUs/1 -> _PDUs_/1  "PDUs"
  _PDUs_/1 -> TCU05/1(TCU05)  "<TCU05>"
  _PDUs_/2 -> TCU03/1(TCU03)  "<TCU03>"
  _PDUs_/3 -> TCU02/1(TCU02)  "<TCU02>"
  _PDUs_/4 -> TCU01/1(TCU01)  "<TCU01>"
  _PDUs_/5 -> BMS01/1(BMS01)  "<BMS01>"
  _PDUs_/6 -> MainController/1(MainController)  "<MainController>"
  _PDUs_/7 -> BMS02/1(BMS02)  "<BMS02>"
  _PDUs_/8 -> TCU04/1(TCU04)  "<TCU04>"

== system DriveSystemControl/Bus Configuration (1) - Out/Simulated ECUs/gitam Controller CAN File 08082024/BMS/RX/PDUs ==
  PDUs : Inport
  TCU04 : Subsystem
  _PDUs_ : BusSelector  OutputSignals=TCU04
  wires:
  PDUs/1 -> _PDUs_/1  "PDUs"
  _PDUs_/1 -> TCU04/1(TCU04)  "<TCU04>"

== system DriveSystemControl/Bus Configuration (1) - Out/Simulated ECUs/gitam Controller CAN File 08082024/IPC/RX/PDUs ==
  PDUs : Inport
  BMS01 : Subsystem
  TCU01 : Subsystem
  TCU03 : Subsystem
  TCU04 : Subsystem
  TCU05 : Subsystem
  _PDUs_ : BusSelector  OutputSignals=TCU05,TCU04,TCU03,TCU01,BMS01
  wires:
  PDUs/1 -> _PDUs_/1  "PDUs"
  _PDUs_/1 -> TCU05/1(TCU05)  "<TCU05>"
  _PDUs_/2 -> TCU04/1(TCU04)  "<TCU04>"
  _PDUs_/3 -> TCU03/1(TCU03)  "<TCU03>"
  _PDUs_/4 -> TCU01/1(TCU01)  "<TCU01>"
  _PDUs_/5 -> BMS01/1(BMS01)  "<BMS01>"

== system DriveSystemControl/Bus Configuration (1) - Out/Simulated ECUs/gitam Controller CAN File 08082024/TCU/RX/PDUs ==
  PDUs : Inport
  BMS02 : Subsystem
  _PDUs_ : BusSelector  OutputSignals=BMS02
  wires:
  PDUs/1 -> _PDUs_/1  "PDUs"
  _PDUs_/1 -> BMS02/1(BMS02)  "<BMS02>"

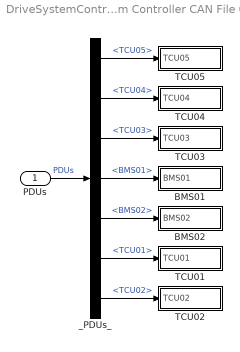
== system DriveSystemControl/Bus Configuration (1) - Out/Simulated ECUs/gitam Controller CAN File 08082024/Telematics/RX/PDUs ==
  PDUs : Inport
  BMS01 : Subsystem
  BMS02 : Subsystem
  TCU01 : Subsystem
  TCU02 : Subsystem
  TCU03 : Subsystem
  TCU04 : Subsystem
  TCU05 : Subsystem
  _PDUs_ : BusSelector  OutputSignals=TCU05,TCU04,TCU03,BMS01,BMS02,TCU01,TCU02
  wires:
  PDUs/1 -> _PDUs_/1  "PDUs"
  _PDUs_/1 -> TCU05/1(TCU05)  "<TCU05>"
  _PDUs_/2 -> TCU04/1(TCU04)  "<TCU04>"
  _PDUs_/3 -> TCU03/1(TCU03)  "<TCU03>"
  _PDUs_/4 -> BMS01/1(BMS01)  "<BMS01>"
  _PDUs_/5 -> BMS02/1(BMS02)  "<BMS02>"
  _PDUs_/6 -> TCU01/1(TCU01)  "<TCU01>"
  _PDUs_/7 -> TCU02/1(TCU02)  "<TCU02>"

== system DriveSystemControl/Bus Configuration (1) - In/Manipulation/gitam Controller CAN File 08082024/WIP/CANChannel/PDUs/BMS01 ==
  _BMS01_ : BusCreator  Inputs=3
  sigBatteryMalfunctionLight : Subsystem
  sigKeyOnIndicator : Subsystem
  sigStateOfCharge : Subsystem
  BMS01 : Outport
  wires:
  _BMS01_/1 -> BMS01/1  "BMS01"
  sigBatteryMalfunctionLight/1(sigBatteryMalfunctionLight) -> _BMS01_/1  "sigBatteryMalfunctionLight"
  sigKeyOnIndicator/1(sigKeyOnIndicator) -> _BMS01_/2  "sigKeyOnIndicator"
  sigStateOfCharge/1(sigStateOfCharge) -> _BMS01_/3  "sigStateOfCharge"

== system DriveSystemControl/Bus Configuration (1) - In/Manipulation/gitam Controller CAN File 08082024/WIP/CANChannel/PDUs/BMS02 ==
  _BMS02_ : BusCreator  Inputs=4
  sigBatteryCurrent : Subsystem
  sigDriveCurrentLimit : Subsystem
  sigRegenCurrentLimit : Subsystem
  sigVehicleModeRequest : Subsystem
  BMS02 : Outport
  wires:
  _BMS02_/1 -> BMS02/1  "BMS02"
  sigVehicleModeRequest/1(sigVehicleModeRequest) -> _BMS02_/1  "sigVehicleModeRequest"
  sigRegenCurrentLimit/1(sigRegenCurrentLimit) -> _BMS02_/2  "sigRegenCurrentLimit"
  sigDriveCurrentLimit/1(sigDriveCurrentLimit) -> _BMS02_/3  "sigDriveCurrentLimit"
  sigBatteryCurrent/1(sigBatteryCurrent) -> _BMS02_/4  "sigBatteryCurrent"

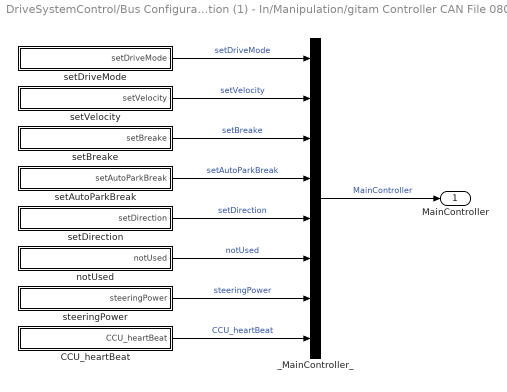
== system DriveSystemControl/Bus Configuration (1) - In/Manipulation/gitam Controller CAN File 08082024/WIP/CANChannel/PDUs/MainController ==
  CCU_heartBeat : Subsystem
  _MainController_ : BusCreator  Inputs=8
  notUsed : Subsystem
  setAutoParkBreak : Subsystem
  setBreake : Subsystem
  setDirection : Subsystem
  setDriveMode : Subsystem
  setVelocity : Subsystem
  steeringPower : Subsystem
  MainController : Outport
  wires:
  _MainController_/1 -> MainController/1  "MainController"
  setDriveMode/1(setDriveMode) -> _MainController_/1  "setDriveMode"
  setVelocity/1(setVelocity) -> _MainController_/2  "setVelocity"
  setBreake/1(setBreake) -> _MainController_/3  "setBreake"
  setAutoParkBreak/1(setAutoParkBreak) -> _MainController_/4  "setAutoParkBreak"
  setDirection/1(setDirection) -> _MainController_/5  "setDirection"
  notUsed/1(notUsed) -> _MainController_/6  "notUsed"
  steeringPower/1(steeringPower) -> _MainController_/7  "steeringPower"
  CCU_heartBeat/1(CCU_heartBeat) -> _MainController_/8  "CCU_heartBeat"

== system DriveSystemControl/Bus Configuration (1) - In/Manipulation/gitam Controller CAN File 08082024/WIP/CANChannel/PDUs/TCU01 ==
  _TCU01_ : BusCreator  Inputs=7
  sigBrake : Subsystem
  sigControllerTemperature : Subsystem
  sigDriveMode : Subsystem
  sigMotorTemperature : Subsystem
  sigRMSCurrent : Subsystem
  sigSpeed : Subsystem
  sigThrottle : Subsystem
  TCU01 : Outport
  wires:
  _TCU01_/1 -> TCU01/1  "TCU01"
  sigBrake/1(sigBrake) -> _TCU01_/1  "sigBrake"
  sigDriveMode/1(sigDriveMode) -> _TCU01_/2  "sigDriveMode"
  sigSpeed/1(sigSpeed) -> _TCU01_/3  "sigSpeed"
  sigThrottle/1(sigThrottle) -> _TCU01_/4  "sigThrottle"
  sigRMSCurrent/1(sigRMSCurrent) -> _TCU01_/5  "sigRMSCurrent"
  sigMotorTemperature/1(sigMotorTemperature) -> _TCU01_/6  "sigMotorTemperature"
  sigControllerTemperature/1(sigControllerTemperature) -> _TCU01_/7  "sigControllerTemperature"

== system DriveSystemControl/Bus Configuration (1) - In/Manipulation/gitam Controller CAN File 08082024/WIP/CANChannel/PDUs/TCU02 ==
  _TCU02_ : BusCreator  Inputs=3
  sigCapacitorVoltage : Subsystem
  sigMotorRPM : Subsystem
  sigOdometer : Subsystem
  TCU02 : Outport
  wires:
  _TCU02_/1 -> TCU02/1  "TCU02"
  sigOdometer/1(sigOdometer) -> _TCU02_/1  "sigOdometer"
  sigCapacitorVoltage/1(sigCapacitorVoltage) -> _TCU02_/2  "sigCapacitorVoltage"
  sigMotorRPM/1(sigMotorRPM) -> _TCU02_/3  "sigMotorRPM"

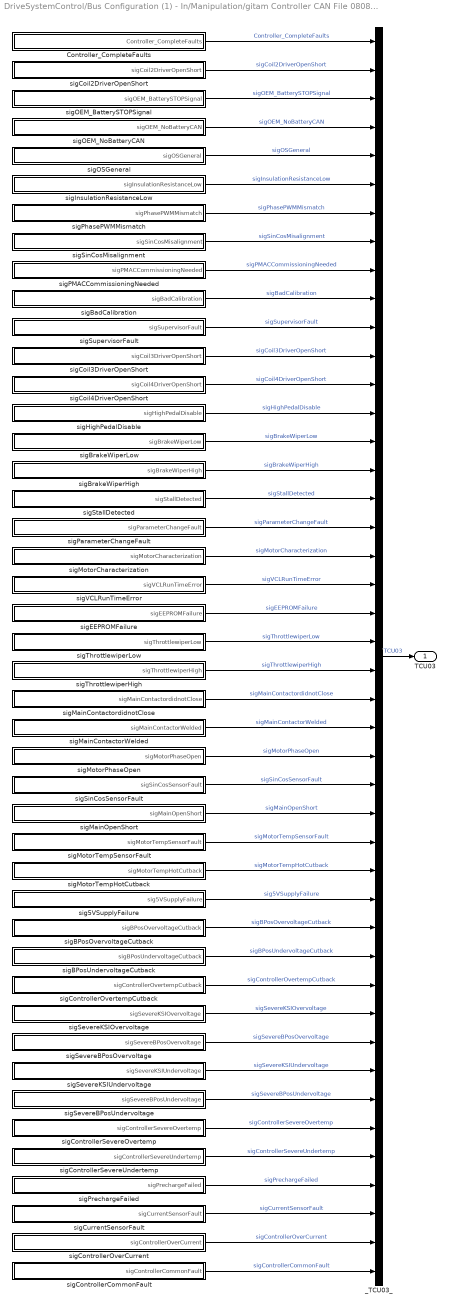
== system DriveSystemControl/Bus Configuration (1) - In/Manipulation/gitam Controller CAN File 08082024/WIP/CANChannel/PDUs/TCU03 ==
  Controller_CompleteFaults : Subsystem
  _TCU03_ : BusCreator  Inputs=44
  sig5VSupplyFailure : Subsystem
  sigBPosOvervoltageCutback : Subsystem
  sigBPosUndervoltageCutback : Subsystem
  sigBadCalibration : Subsystem
  sigBrakeWiperHigh : Subsystem
  sigBrakeWiperLow : Subsystem
  sigCoil2DriverOpenShort : Subsystem
  sigCoil3DriverOpenShort : Subsystem
  sigCoil4DriverOpenShort : Subsystem
  sigControllerCommonFault : Subsystem
  sigControllerOverCurrent : Subsystem
  sigControllerOvertempCutback : Subsystem
  sigControllerSevereOvertemp : Subsystem
  sigControllerSevereUndertemp : Subsystem
  sigCurrentSensorFault : Subsystem
  sigEEPROMFailure : Subsystem
  sigHighPedalDisable : Subsystem
  sigInsulationResistanceLow : Subsystem
  sigMainContactorWelded : Subsystem
  sigMainContactordidnotClose : Subsystem
  sigMainOpenShort : Subsystem
  sigMotorCharacterization : Subsystem
  sigMotorPhaseOpen : Subsystem
  sigMotorTempHotCutback : Subsystem
  sigMotorTempSensorFault : Subsystem
  sigOEM_BatterySTOPSignal : Subsystem
  sigOEM_NoBatteryCAN : Subsystem
  sigOSGeneral : Subsystem
  sigPMACCommissioningNeeded : Subsystem
  sigParameterChangeFault : Subsystem
  sigPhasePWMMismatch : Subsystem
  sigPrechargeFailed : Subsystem
  sigSevereBPosOvervoltage : Subsystem
  sigSevereBPosUndervoltage : Subsystem
  sigSevereKSIOvervoltage : Subsystem
  sigSevereKSIUndervoltage : Subsystem
  sigSinCosMisalignment : Subsystem
  sigSinCosSensorFault : Subsystem
  sigStallDetected : Subsystem
  sigSupervisorFault : Subsystem
  sigThrottlewiperHigh : Subsystem
  sigThrottlewiperLow : Subsystem
  sigVCLRunTimeError : Subsystem
  TCU03 : Outport
  wires:
  _TCU03_/1 -> TCU03/1  "TCU03"
  Controller_CompleteFaults/1(Controller_CompleteFaults) -> _TCU03_/1  "Controller_CompleteFaults"
  sigCoil2DriverOpenShort/1(sigCoil2DriverOpenShort) -> _TCU03_/2  "sigCoil2DriverOpenShort"
  sigOEM_BatterySTOPSignal/1(sigOEM_BatterySTOPSignal) -> _TCU03_/3  "sigOEM_BatterySTOPSignal"
  sigOEM_NoBatteryCAN/1(sigOEM_NoBatteryCAN) -> _TCU03_/4  "sigOEM_NoBatteryCAN"
  sigOSGeneral/1(sigOSGeneral) -> _TCU03_/5  "sigOSGeneral"
  sigInsulationResistanceLow/1(sigInsulationResistanceLow) -> _TCU03_/6  "sigInsulationResistanceLow"
  sigPhasePWMMismatch/1(sigPhasePWMMismatch) -> _TCU03_/7  "sigPhasePWMMismatch"
  sigSinCosMisalignment/1(sigSinCosMisalignment) -> _TCU03_/8  "sigSinCosMisalignment"
  sigPMACCommissioningNeeded/1(sigPMACCommissioningNeeded) -> _TCU03_/9  "sigPMACCommissioningNeeded"
  sigBadCalibration/1(sigBadCalibration) -> _TCU03_/10  "sigBadCalibration"
  sigSupervisorFault/1(sigSupervisorFault) -> _TCU03_/11  "sigSupervisorFault"
  sigCoil3DriverOpenShort/1(sigCoil3DriverOpenShort) -> _TCU03_/12  "sigCoil3DriverOpenShort"
  sigCoil4DriverOpenShort/1(sigCoil4DriverOpenShort) -> _TCU03_/13  "sigCoil4DriverOpenShort"
  sigHighPedalDisable/1(sigHighPedalDisable) -> _TCU03_/14  "sigHighPedalDisable"
  sigBrakeWiperLow/1(sigBrakeWiperLow) -> _TCU03_/15  "sigBrakeWiperLow"
  sigBrakeWiperHigh/1(sigBrakeWiperHigh) -> _TCU03_/16  "sigBrakeWiperHigh"
  sigStallDetected/1(sigStallDetected) -> _TCU03_/17  "sigStallDetected"
  sigParameterChangeFault/1(sigParameterChangeFault) -> _TCU03_/18  "sigParameterChangeFault"
  sigMotorCharacterization/1(sigMotorCharacterization) -> _TCU03_/19  "sigMotorCharacterization"
  sigVCLRunTimeError/1(sigVCLRunTimeError) -> _TCU03_/20  "sigVCLRunTimeError"
  sigEEPROMFailure/1(sigEEPROMFailure) -> _TCU03_/21  "sigEEPROMFailure"
  sigThrottlewiperLow/1(sigThrottlewiperLow) -> _TCU03_/22  "sigThrottlewiperLow"
  sigThrottlewiperHigh/1(sigThrottlewiperHigh) -> _TCU03_/23  "sigThrottlewiperHigh"
  sigMainContactordidnotClose/1(sigMainContactordidnotClose) -> _TCU03_/24  "sigMainContactordidnotClose"
  sigMainContactorWelded/1(sigMainContactorWelded) -> _TCU03_/25  "sigMainContactorWelded"
  sigMotorPhaseOpen/1(sigMotorPhaseOpen) -> _TCU03_/26  "sigMotorPhaseOpen"
  sigSinCosSensorFault/1(sigSinCosSensorFault) -> _TCU03_/27  "sigSinCosSensorFault"
  sigMainOpenShort/1(sigMainOpenShort) -> _TCU03_/28  "sigMainOpenShort"
  sigMotorTempSensorFault/1(sigMotorTempSensorFault) -> _TCU03_/29  "sigMotorTempSensorFault"
  sigMotorTempHotCutback/1(sigMotorTempHotCutback) -> _TCU03_/30  "sigMotorTempHotCutback"
  sig5VSupplyFailure/1(sig5VSupplyFailure) -> _TCU03_/31  "sig5VSupplyFailure"
  sigBPosOvervoltageCutback/1(sigBPosOvervoltageCutback) -> _TCU03_/32  "sigBPosOvervoltageCutback"
  sigBPosUndervoltageCutback/1(sigBPosUndervoltageCutback) -> _TCU03_/33  "sigBPosUndervoltageCutback"
  sigControllerOvertempCutback/1(sigControllerOvertempCutback) -> _TCU03_/34  "sigControllerOvertempCutback"
  sigSevereKSIOvervoltage/1(sigSevereKSIOvervoltage) -> _TCU03_/35  "sigSevereKSIOvervoltage"
  sigSevereBPosOvervoltage/1(sigSevereBPosOvervoltage) -> _TCU03_/36  "sigSevereBPosOvervoltage"
  sigSevereKSIUndervoltage/1(sigSevereKSIUndervoltage) -> _TCU03_/37  "sigSevereKSIUndervoltage"
  sigSevereBPosUndervoltage/1(sigSevereBPosUndervoltage) -> _TCU03_/38  "sigSevereBPosUndervoltage"
  sigControllerSevereOvertemp/1(sigControllerSevereOvertemp) -> _TCU03_/39  "sigControllerSevereOvertemp"
  sigControllerSevereUndertemp/1(sigControllerSevereUndertemp) -> _TCU03_/40  "sigControllerSevereUndertemp"
  sigPrechargeFailed/1(sigPrechargeFailed) -> _TCU03_/41  "sigPrechargeFailed"
  sigCurrentSensorFault/1(sigCurrentSensorFault) -> _TCU03_/42  "sigCurrentSensorFault"
  sigControllerOverCurrent/1(sigControllerOverCurrent) -> _TCU03_/43  "sigControllerOverCurrent"
  sigControllerCommonFault/1(sigControllerCommonFault) -> _TCU03_/44  "sigControllerCommonFault"

== system DriveSystemControl/Bus Configuration (1) - In/Manipulation/gitam Controller CAN File 08082024/WIP/CANChannel/PDUs/TCU04 ==
  _TCU04_ : BusCreator  Inputs=5
  sigMCU5_DriveMode : Subsystem
  sigMCU5_Efficiency : Subsystem
  sigMCU5_Hillhold : Subsystem
  sigMCU5_RegenFlag : Subsystem
  sigMCU5_Speed : Subsystem
  TCU04 : Outport
  wires:
  _TCU04_/1 -> TCU04/1  "TCU04"
  sigMCU5_Efficiency/1(sigMCU5_Efficiency) -> _TCU04_/1  "sigMCU5_Efficiency"
  sigMCU5_Hillhold/1(sigMCU5_Hillhold) -> _TCU04_/2  "sigMCU5_Hillhold"
  sigMCU5_Speed/1(sigMCU5_Speed) -> _TCU04_/3  "sigMCU5_Speed"
  sigMCU5_RegenFlag/1(sigMCU5_RegenFlag) -> _TCU04_/4  "sigMCU5_RegenFlag"
  sigMCU5_DriveMode/1(sigMCU5_DriveMode) -> _TCU04_/5  "sigMCU5_DriveMode"

== system DriveSystemControl/Bus Configuration (1) - In/Manipulation/gitam Controller CAN File 08082024/WIP/CANChannel/PDUs/TCU05 ==
  _TCU05_ : BusCreator  Inputs=1
  sigMCU6_Odometer : Subsystem
  TCU05 : Outport
  wires:
  _TCU05_/1 -> TCU05/1  "TCU05"
  sigMCU6_Odometer/1(sigMCU6_Odometer) -> _TCU05_/1  "sigMCU6_Odometer"

== system DriveSystemControl/Bus Configuration (1) - In/Simulated ECUs/gitam Controller CAN File 08082024/BMS/TX/PDUs/BMS01 ==
  _BMS01_ : BusCreator  Inputs=3
  sigBatteryMalfunctionLight : Subsystem
  sigKeyOnIndicator : Subsystem
  sigStateOfCharge : Subsystem
  BMS01 : Outport
  wires:
  _BMS01_/1 -> BMS01/1  "BMS01"
  sigBatteryMalfunctionLight/1(sigBatteryMalfunctionLight) -> _BMS01_/1  "sigBatteryMalfunctionLight"
  sigKeyOnIndicator/1(sigKeyOnIndicator) -> _BMS01_/2  "sigKeyOnIndicator"
  sigStateOfCharge/1(sigStateOfCharge) -> _BMS01_/3  "sigStateOfCharge"
